simulink model "sl2ge_hyperloop"  (R2014a)
settings: Solver=FixedStepDiscrete  StartTime=startTime  StopTime=stopTime  FixedStep=0.025  MaxStep=0.1  RelTol=1e-3
values from neighbouring files (symbols this model uses):
  dactOffset = 0    [main_sl2ge.m]
  latOffset = offsetNSinMeters/110958.98    (= 0.0001802467903)    [main_sl2ge.m]
  pillarSpacing = 30    [main_sl2ge.m]
  startTime = 0    [main_sl2ge.m]    (also in sl2ge_multiple.m = evalin('base','startTime'))
  stopTime = logsout.getElement('dact').Values.Time(end)    [main_sl2ge.m]
undefined symbols (not defined in the file or in its folder): camHt_1LVal, camHt_1UVal, Chassis, getLOatTime, logsout, numPillars, sigbuilder_block, z_accel, z_dist, z_elevTube, z_height
undefined symbols (not defined in the file): camHt_1LTh, camHt_1UTh, camHt_2LTh, camHt_2UTh
libraries: simulink x10, realtime_pacer_lib x1, vrlib x1
settings Model: Creator=Administrator  LastModifiedBy=mbrauer
settings DataIOCC: SignalLoggingSaveFormat=ModelDataLogs  SignalLogging=off
settings OptimizationCC: ExpressionDepthLimit=2147483647
settings DebuggingCC: UnderspecifiedInitializationDetection=Classic  InheritedTsInSrcMsg=none  FcnCallInpInsideContextMsg=EnableAllAsWarning  StateNameClashWarn=warning
settings RTWCC: ProcessScript=grt_make_rtw_hook

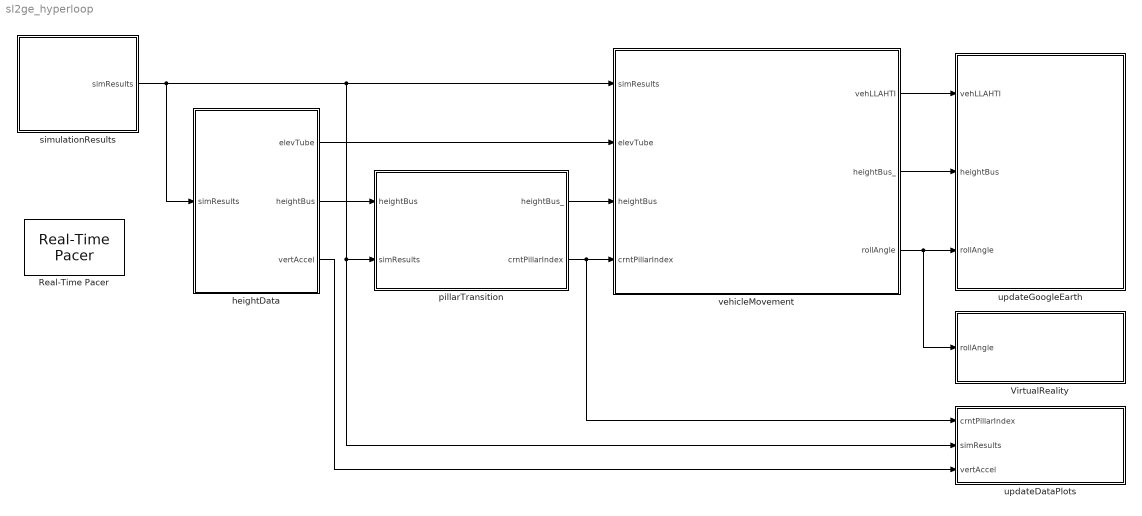
== system sl2ge_hyperloop ==
  Real-Time Pacer : realtime_pacer_lib/Real-Time Pacer  simTimePerRealTime=0.125
  VirtualReality : Subsystem
  heightData : Subsystem
  pillarTransition : Subsystem
  simulationResults : Subsystem
  updateDataPlots : Subsystem
  updateGoogleEarth : Subsystem
  vehicleMovement : Subsystem
  wires:
  heightData/1(elevTube) -> vehicleMovement/2(elevTube)
  pillarTransition/2(crntPillarIndex) -> vehicleMovement/4(crntPillarIndex), updateDataPlots/1(crntPillarIndex)
  vehicleMovement/3(rollAngle) -> updateGoogleEarth/3(rollAngle), VirtualReality/1(rollAngle)
  heightData/3(vertAccel) -> updateDataPlots/3(vertAccel)
  heightData/2(heightBus) -> pillarTransition/1(heightBus)
  pillarTransition/1(heightBus_) -> vehicleMovement/3(heightBus)
  vehicleMovement/2(heightBus_) -> updateGoogleEarth/2(heightBus)
  vehicleMovement/1(vehLLAHTI) -> updateGoogleEarth/1(vehLLAHTI)
  simulationResults/1(simResults) -> vehicleMovement/1(simResults), updateDataPlots/2(simResults), pillarTransition/2(simResults), heightData/1(simResults)

== system sl2ge_hyperloop/VirtualReality ==
  rollAngle : Inport
  CenterOfRotation : Constant  Value=[-1.54/2 sqrt(Chassis.TubeRadius^2-(1.54/2)^2) 0]'  SampleTime=-1
  Constant : Constant  Value=[0 0 1]'  SampleTime=-1
  Gain6 : Gain  Gain=-1
  VR Sink : vrlib/VR Sink  InstantiateOnLoad=on  SampleTime=-1  ViewEnable=on  RemoteChange=off  RemoteView=off  FieldsWritten=HyperPod.center.3.1.1.double#HyperPod.rotation.4.1.1.double  WorldFileName=hyperLoopPod3DTubeIso.wrl  WorldDescription=Simulink 3D Animation : Front View of Pod  AutoView=off  VideoDimensions=[]  AllowVariableSize=off
  Vector Concatenate1 : Concatenate
  wires:
  Gain6/1 -> Vector Concatenate1/2
  Constant/1 -> Vector Concatenate1/1
  CenterOfRotation/1 -> VR Sink/1
  Vector Concatenate1/1 -> VR Sink/2
  rollAngle/1 -> Gain6/1

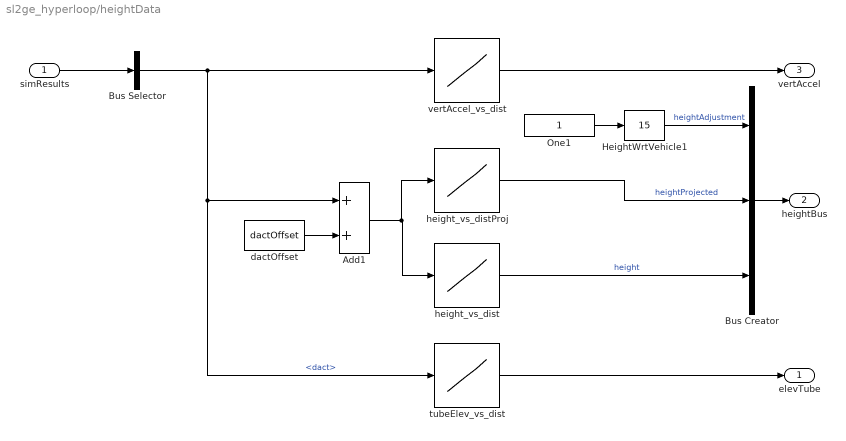
== system sl2ge_hyperloop/heightData ==
  simResults : Inport
  Add1 : Sum
  Bus Creator : BusCreator  Inputs=3
  Bus Selector : BusSelector  OutputSignals=dact
  HeightWrtVehicle1 : simulink/Math Operations/Slider Gain  low=-10  gain=15  high=30
  One1 : Constant  VectorParams1D=off
  dactOffset : Constant  Value=dactOffset
  height_vs_dist : Lookup_n-D  NumberOfTableDimensions=1  BreakpointsForDimension1=z_dist  BeginIndexSearchUsingPreviousIndexResult=on  Table=z_height  ExtrapMethod=Clip  InternalRulePriority=Speed  RndMeth=Simplest  InputSameDT=on
  height_vs_distProj : Lookup_n-D  NumberOfTableDimensions=1  BreakpointsForDimension1=z_dist-200  BeginIndexSearchUsingPreviousIndexResult=on  Table=z_height  ExtrapMethod=Clip  UseLastTableValue=on  InternalRulePriority=Speed  RndMeth=Simplest  InputSameDT=on
  tubeElev_vs_dist : Lookup_n-D  NumberOfTableDimensions=1  BreakpointsForDimension1=z_dist  BeginIndexSearchUsingPreviousIndexResult=on  Table=z_elevTube  InternalRulePriority=Speed  RndMeth=Simplest  InputSameDT=on
  vertAccel_vs_dist : Lookup_n-D  NumberOfTableDimensions=1  BreakpointsForDimension1=z_dist  BeginIndexSearchUsingPreviousIndexResult=on  Table=z_accel  ExtrapMethod=Clip  UseLastTableValue=on  InternalRulePriority=Speed  RndMeth=Simplest  InputSameDT=on
  elevTube : Outport
  heightBus : Outport  Port=2
  vertAccel : Outport  Port=3
  wires:
  height_vs_distProj/1 -> Bus Creator/2  "heightProjected"
  vertAccel_vs_dist/1 -> vertAccel/1
  height_vs_dist/1 -> Bus Creator/3  "height"
  tubeElev_vs_dist/1 -> elevTube/1
  Bus Selector/1 -> vertAccel_vs_dist/1, tubeElev_vs_dist/1, Add1/1  "<dact>"
  dactOffset/1 -> Add1/2
  Add1/1 -> height_vs_distProj/1, height_vs_dist/1
  One1/1 -> HeightWrtVehicle1/1
  HeightWrtVehicle1/1 -> Bus Creator/1  "heightAdjustment"
  Bus Creator/1 -> heightBus/1
  simResults/1 -> Bus Selector/1

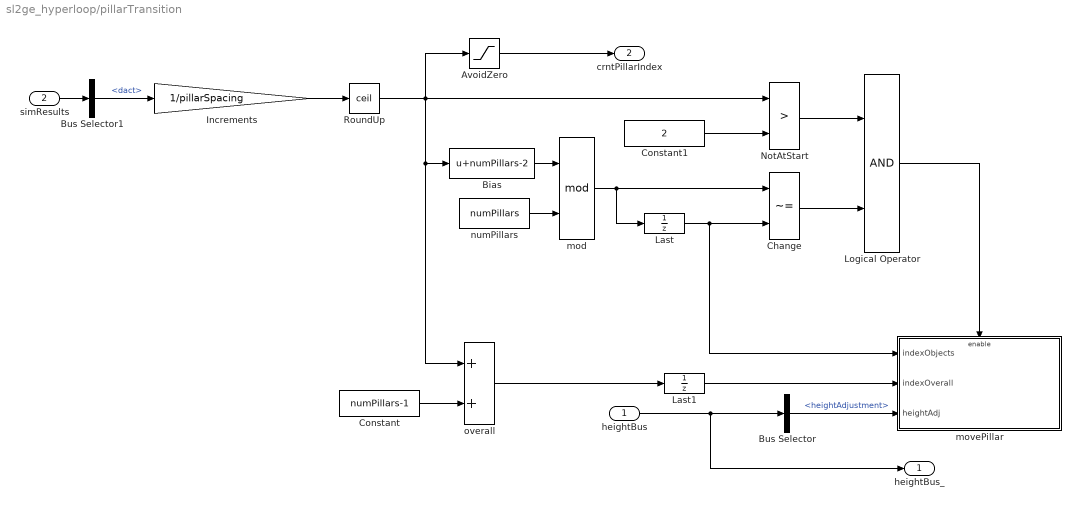
== system sl2ge_hyperloop/pillarTransition ==
  heightBus : Inport
  simResults : Inport  Port=2
  AvoidZero : Saturate  UpperLimit=inf  LowerLimit=1
  Bias : Bias  Bias=numPillars-2
  Bus Selector : BusSelector  OutputSignals=heightAdjustment
  Bus Selector1 : BusSelector  OutputSignals=dact
  Change : RelationalOperator  Operator=~=  OutDataTypeStr=boolean
  Constant : Constant  Value=numPillars-1
  Constant1 : Constant  Value=2
  Increments : Gain  Gain=1/pillarSpacing
  Last : UnitDelay  SampleTime=-1
  Last1 : UnitDelay  InitialCondition=1  SampleTime=-1
  Logical Operator : Logic  AllPortsSameDT=off  OutDataTypeStr=boolean
  NotAtStart : RelationalOperator  Operator=>  OutDataTypeStr=boolean
  RoundUp : Rounding  Operator=ceil
  mod : Math  Operator=mod  SaturateOnIntegerOverflow=on
  movePillar : Subsystem  TreatAsAtomicUnit=on
  numPillars : Constant  Value=numPillars
  overall : Sum
  heightBus_ : Outport
  crntPillarIndex : Outport  Port=2
  wires:
  Bus Selector1/1 -> Increments/1  "<dact>"
  Increments/1 -> RoundUp/1
  mod/1 -> Change/1, Last/1
  numPillars/1 -> mod/2
  Last/1 -> movePillar/1(indexObjects), Change/2
  overall/1 -> Last1/1
  Constant/1 -> overall/2
  Change/1 -> Logical Operator/2
  NotAtStart/1 -> Logical Operator/1
  Constant1/1 -> NotAtStart/2
  Logical Operator/1 -> movePillar/Enable
  Bias/1 -> mod/1
  RoundUp/1 -> AvoidZero/1, overall/1, Bias/1, NotAtStart/1
  Last1/1 -> movePillar/2(indexOverall)
  AvoidZero/1 -> crntPillarIndex/1
  heightBus/1 -> Bus Selector/1, heightBus_/1
  Bus Selector/1 -> movePillar/3(heightAdj)  "<heightAdjustment>"
  simResults/1 -> Bus Selector1/1

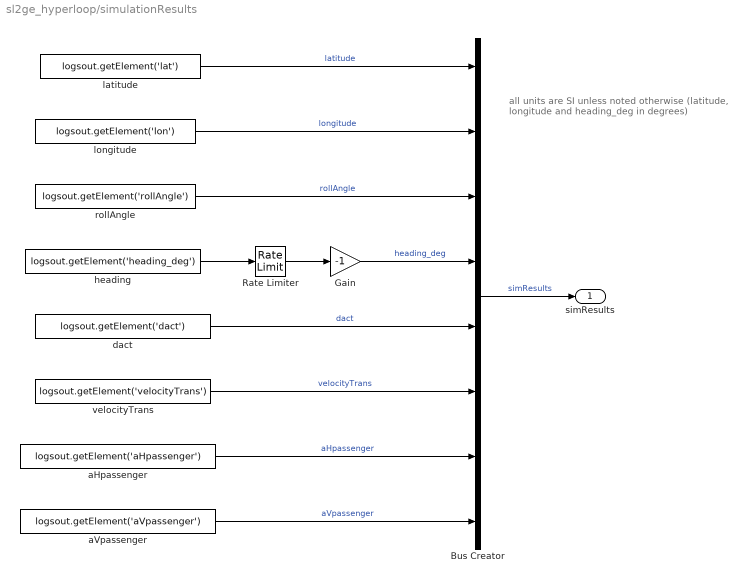
== system sl2ge_hyperloop/simulationResults ==
  note: all units are SI unless noted otherwise
      | (latitude, longitude and heading_deg in degrees)
  Bus Creator : BusCreator  Inputs=8
  Gain : Gain  Gain=-1
  Rate Limiter : RateLimiter  RisingSlewLimit=5  FallingSlewLimit=-5  SampleTimeMode=inherited  InitialCondition=getLOatTime(logsout, 'heading_deg', startTime)
  aHpassenger : FromWorkspace  VariableName=logsout.getElement('aHpassenger')
  aVpassenger : FromWorkspace  VariableName=logsout.getElement('aVpassenger')
  dact : FromWorkspace  VariableName=logsout.getElement('dact')
  heading : FromWorkspace  VariableName=logsout.getElement('heading_deg')
  latitude : FromWorkspace  VariableName=logsout.getElement('lat')
  longitude : FromWorkspace  VariableName=logsout.getElement('lon')
  rollAngle : FromWorkspace  VariableName=logsout.getElement('rollAngle')
  velocityTrans : FromWorkspace  VariableName=logsout.getElement('velocityTrans')
  simResults : Outport
  wires:
  Rate Limiter/1 -> Gain/1
  heading/1 -> Rate Limiter/1
  latitude/1 -> Bus Creator/1  "latitude"
  longitude/1 -> Bus Creator/2  "longitude"
  rollAngle/1 -> Bus Creator/3  "rollAngle"
  Gain/1 -> Bus Creator/4  "heading_deg"
  aHpassenger/1 -> Bus Creator/7  "aHpassenger"
  velocityTrans/1 -> Bus Creator/6  "velocityTrans"
  aVpassenger/1 -> Bus Creator/8  "aVpassenger"
  dact/1 -> Bus Creator/5  "dact"
  Bus Creator/1 -> simResults/1  "simResults"

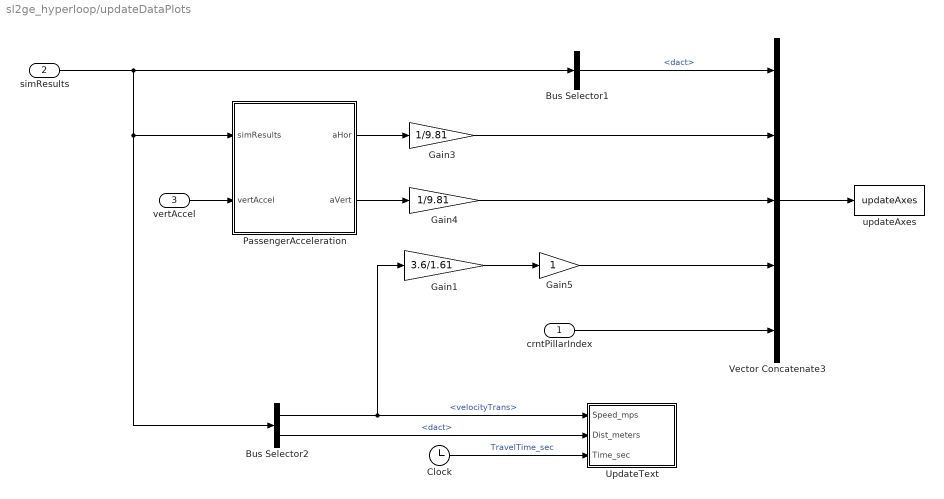
== system sl2ge_hyperloop/updateDataPlots ==
  crntPillarIndex : Inport
  simResults : Inport  Port=2
  vertAccel : Inport  Port=3
  Bus Selector1 : BusSelector  OutputSignals=dact
  Bus Selector2 : BusSelector  OutputSignals=velocityTrans,dact
  Clock : Clock
  Gain1 : Gain  Gain=3.6/1.61
  Gain3 : Gain  Gain=1/9.81
  Gain4 : Gain  Gain=1/9.81
  Gain5 : Gain
  PassengerAcceleration : Subsystem
  UpdateText : Subsystem
  Vector Concatenate3 : Concatenate  NumInputs=5  Mode=Multidimensional array  ConcatenateDimension=2
  updateAxes : MATLABFcn  MATLABFcn=updateAxes  OutputDimensions=0
  wires:
  Gain5/1 -> Vector Concatenate3/4
  Vector Concatenate3/1 -> updateAxes/1
  Gain3/1 -> Vector Concatenate3/2
  Gain4/1 -> Vector Concatenate3/3
  Gain1/1 -> Gain5/1
  Bus Selector2/1 -> Gain1/1, UpdateText/1(Speed_mps)  "<velocityTrans>"
  crntPillarIndex/1 -> Vector Concatenate3/5
  Bus Selector1/1 -> Vector Concatenate3/1  "<dact>"
  Clock/1 -> UpdateText/3(Time_sec)  "TravelTime_sec"
  PassengerAcceleration/1(aHor) -> Gain3/1
  PassengerAcceleration/2(aVert) -> Gain4/1
  vertAccel/1 -> PassengerAcceleration/2(vertAccel)
  simResults/1 -> PassengerAcceleration/1(simResults), Bus Selector2/1, Bus Selector1/1
  Bus Selector2/2 -> UpdateText/2(Dist_meters)  "<dact>"

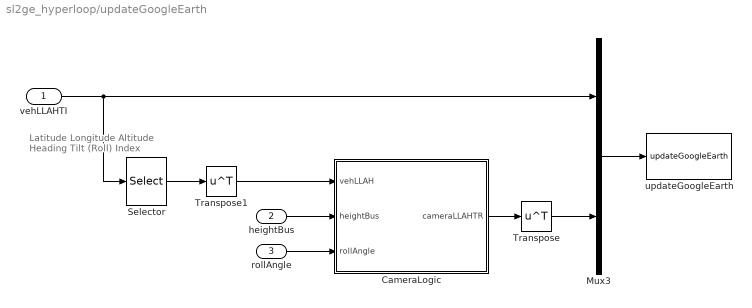
== system sl2ge_hyperloop/updateGoogleEarth ==
  note: Latitude
      | Longitude
      | Altitude
      | Heading
      | Tilt (Roll)
      | Index
  vehLLAHTI : Inport
  heightBus : Inport  Port=2
  rollAngle : Inport  Port=3
  CameraLogic : Subsystem
  Mux3 : Mux  Inputs=2
  Selector : Selector  InputPortWidth=6  Indices=[1 2 3 4]
  Transpose : Math  Operator=transpose  SaturateOnIntegerOverflow=on
  Transpose1 : Math  Operator=transpose  SaturateOnIntegerOverflow=on
  updateGoogleEarth : MATLABFcn  MATLABFcn=updateGoogleEarth  OutputDimensions=0
  wires:
  Selector/1 -> Transpose1/1
  Transpose/1 -> Mux3/2
  vehLLAHTI/1 -> Selector/1, Mux3/1
  Mux3/1 -> updateGoogleEarth/1
  Transpose1/1 -> CameraLogic/1(vehLLAH)
  heightBus/1 -> CameraLogic/2(heightBus)
  rollAngle/1 -> CameraLogic/3(rollAngle)
  CameraLogic/1(cameraLLAHTR) -> Transpose/1

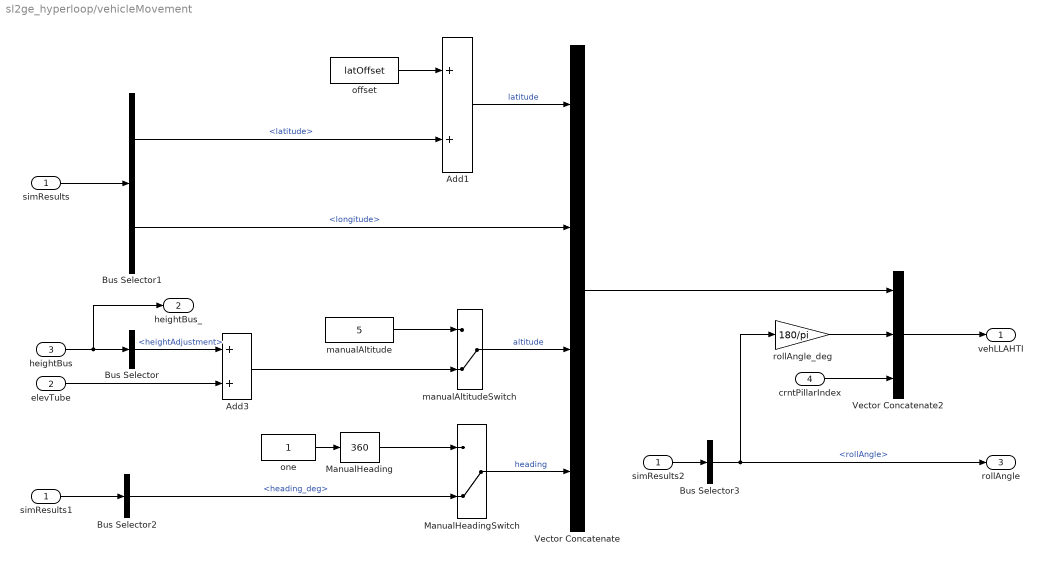
== system sl2ge_hyperloop/vehicleMovement ==
  simResults : Inport
  elevTube : Inport  Port=2
  heightBus : Inport  Port=3
  crntPillarIndex : Inport  Port=4
  Add1 : Sum
  Add3 : Sum
  Bus Selector : BusSelector  OutputSignals=heightAdjustment
  Bus Selector1 : BusSelector  OutputSignals=latitude,longitude
  Bus Selector2 : BusSelector  OutputSignals=heading_deg
  Bus Selector3 : BusSelector  OutputSignals=rollAngle
  ManualHeading : simulink/Math Operations/Slider Gain  low=-360  gain=360  high=360
  ManualHeadingSwitch : ManualSwitch  CurrentSetting=0
  Vector Concatenate : Concatenate  NumInputs=4  Mode=Multidimensional array  ConcatenateDimension=2
  Vector Concatenate2 : Concatenate  NumInputs=3  ConcatenateDimension=2
  manualAltitude : Constant  Value=5  VectorParams1D=off
  manualAltitudeSwitch : ManualSwitch  CurrentSetting=0
  offset : Constant  Value=latOffset  VectorParams1D=off
  one : Constant  VectorParams1D=off
  rollAngle_deg : Gain  Gain=180/pi
  simResults1 : InportShadow
  simResults2 : InportShadow
  vehLLAHTI : Outport
  heightBus_ : Outport  Port=2
  rollAngle : Outport  Port=3
  wires:
  Vector Concatenate2/1 -> vehLLAHTI/1
  rollAngle_deg/1 -> Vector Concatenate2/2
  Vector Concatenate/1 -> Vector Concatenate2/1
  Add3/1 -> manualAltitudeSwitch/2
  heightBus/1 -> Bus Selector/1, heightBus_/1
  manualAltitudeSwitch/1 -> Vector Concatenate/3  "altitude"
  manualAltitude/1 -> manualAltitudeSwitch/1
  Bus Selector2/1 -> ManualHeadingSwitch/2  "<heading_deg>"
  one/1 -> ManualHeading/1
  ManualHeadingSwitch/1 -> Vector Concatenate/4  "heading"
  Bus Selector1/2 -> Vector Concatenate/2  "<longitude>"
  crntPillarIndex/1 -> Vector Concatenate2/3
  Bus Selector1/1 -> Add1/2  "<latitude>"
  Add1/1 -> Vector Concatenate/1  "latitude"
  offset/1 -> Add1/1
  Bus Selector/1 -> Add3/1  "<heightAdjustment>"
  elevTube/1 -> Add3/2
  ManualHeading/1 -> ManualHeadingSwitch/1
  simResults/1 -> Bus Selector1/1
  simResults1/1 -> Bus Selector2/1
  simResults2/1 -> Bus Selector3/1
  Bus Selector3/1 -> rollAngle_deg/1, rollAngle/1  "<rollAngle>"

== system sl2ge_hyperloop/pillarTransition/movePillar ==
  indexObjects : Inport
  indexOverall : Inport  Port=2
  heightAdj : Inport  Port=3
  Enable : EnablePort  StatesWhenEnabling=reset
  Mux : Mux  Inputs=3
  updatePillar : MATLABFcn  MATLABFcn=updatePillars  OutputDimensions=0
  wires:
  indexObjects/1 -> Mux/1
  indexOverall/1 -> Mux/2
  Mux/1 -> updatePillar/1
  heightAdj/1 -> Mux/3

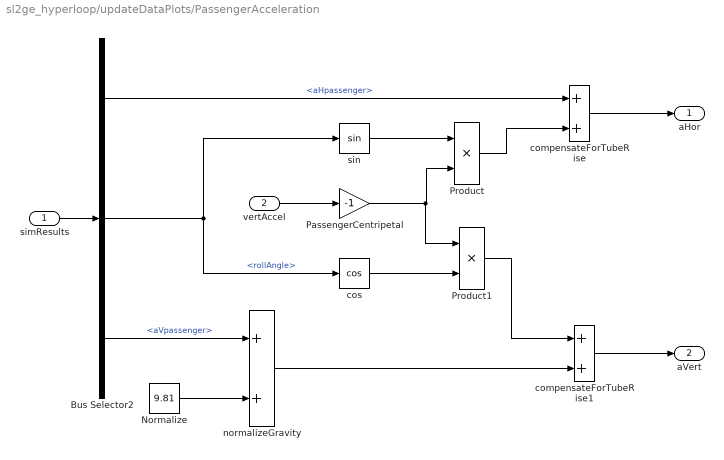
== system sl2ge_hyperloop/updateDataPlots/PassengerAcceleration ==
  simResults : Inport
  vertAccel : Inport  Port=2
  Bus Selector2 : BusSelector  OutputSignals=aHpassenger,rollAngle,aVpassenger
  Normalize : Constant  Value=9.81
  PassengerCentripetal : Gain  Gain=-1
  Product : Product
  Product1 : Product
  compensateForTubeRise : Sum
  compensateForTubeRise1 : Sum
  cos : Trigonometry  Operator=cos
  normalizeGravity : Sum
  sin : Trigonometry
  aHor : Outport
  aVert : Outport  Port=2
  wires:
  Bus Selector2/3 -> normalizeGravity/1  "<aVpassenger>"
  Normalize/1 -> normalizeGravity/2
  Bus Selector2/2 -> cos/1, sin/1  "<rollAngle>"
  sin/1 -> Product/1
  cos/1 -> Product1/2
  vertAccel/1 -> PassengerCentripetal/1
  compensateForTubeRise/1 -> aHor/1
  Bus Selector2/1 -> compensateForTubeRise/1  "<aHpassenger>"
  compensateForTubeRise1/1 -> aVert/1
  normalizeGravity/1 -> compensateForTubeRise1/2
  Product1/1 -> compensateForTubeRise1/1
  Product/1 -> compensateForTubeRise/2
  PassengerCentripetal/1 -> Product1/1, Product/2
  simResults/1 -> Bus Selector2/1

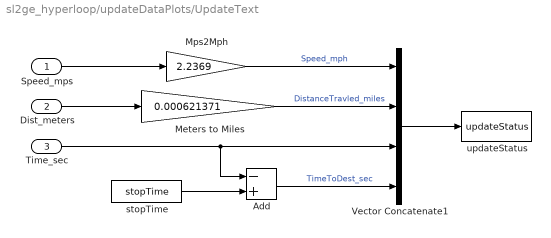
== system sl2ge_hyperloop/updateDataPlots/UpdateText ==
  Speed_mps : Inport
  Dist_meters : Inport  Port=2
  Time_sec : Inport  Port=3
  Add : Sum  Inputs=-+
  Meters to Miles : Gain  Gain=0.000621371
  Mps2Mph : Gain  Gain=2.2369
  Vector Concatenate1 : Concatenate  NumInputs=4  Mode=Multidimensional array  ConcatenateDimension=2
  stopTime : Constant  Value=stopTime
  updateStatus : MATLABFcn  MATLABFcn=updateStatus  OutputDimensions=0
  wires:
  Dist_meters/1 -> Meters to Miles/1
  Vector Concatenate1/1 -> updateStatus/1
  Mps2Mph/1 -> Vector Concatenate1/1  "Speed_mph"
  Meters to Miles/1 -> Vector Concatenate1/2  "DistanceTravled_miles"
  Time_sec/1 -> Vector Concatenate1/3, Add/1
  stopTime/1 -> Add/2
  Add/1 -> Vector Concatenate1/4  "TimeToDest_sec"
  Speed_mps/1 -> Mps2Mph/1

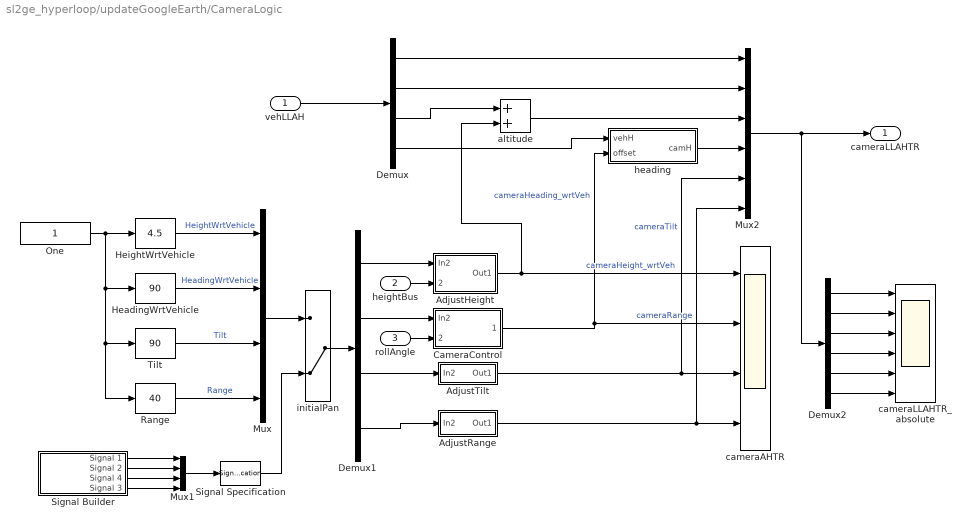
== system sl2ge_hyperloop/updateGoogleEarth/CameraLogic ==
  vehLLAH : Inport
  heightBus : Inport  Port=2
  rollAngle : Inport  Port=3
  AdjustHeight : Subsystem
  AdjustRange : Subsystem
  AdjustTilt : Subsystem
  CameraControl : Subsystem
  Demux : Demux
  Demux1 : Demux
  Demux2 : Demux  Outputs=6
  HeadingWrtVehicle : simulink/Math Operations/Slider Gain  low=65  gain=90  high=115
  HeightWrtVehicle : simulink/Math Operations/Slider Gain  low=0  gain=4.5  high=30
  Mux : Mux
  Mux1 : Mux
  Mux2 : Mux  Inputs=6
  One : Constant  VectorParams1D=off
  Range : simulink/Math Operations/Slider Gain  low=20  gain=40  high=60
  Signal Builder : Subsystem  Tag=STV Subsys  LoadFcn=sigbuilder_block('load');  StartFcn=sigbuilder_block('start');  StopFcn=sigbuilder_block('stop');  ClipboardFcn=sigbuilder_block('clipboard');  mask(Sigbuilder block){}
      mask help: Simulink:masks:SigbuilderBlock_MD
      mask init:
      | if ~strcmp(get_param(bdroot(gcbh),'SimulationStatus'),'stopped') tuvar = sigbuilder_block('maskInit'); end
      settings: CopyFcn=sigbuilder_block('copy');  DeleteFcn=sigbuilder_block('delete');  ModelCloseFcn=sigbuilder_block('modelClose');  PreSaveFcn=sigbuilder_block('preSave');  PauseFcn=sigbuilder_block('pause');  ContinueFcn=sigbuilder_block('continue');  NameChangeFcn=sigbuilder_block('namechange');  OpenFcn=sigbuilder_block('open',[679.5 100.5 550.5 399.75 ]);  CloseFcn=sigbuilder_block('close');
      mask Display: plot(0, 0, 100, 100,[2, 2, 32, 32, 2], [68, 8, 8, 68, 68],[32, 2], [38, 38], [32, 19, 2],[53, 60, 44], [32, 17, 17, 2],[16, 16, 31, 31]);txt = getActiveGroup(gcbh);text(2, 100, txt,'verticalAlignment', 'top');
  Signal Specification : SignalSpecification  SampleTime=0.025
  Tilt : simulink/Math Operations/Slider Gain  low=0  gain=90  high=180
  altitude : Sum
  cameraAHTR : Scope  NumInputPorts=4
      settings: YMin=1.8~35~90~15  YMax=3~70~90~15
  cameraLLAHTR_absolute : Scope  NumInputPorts=6
      settings: YMin=-5~-5~-5~-5~-5~-5  YMax=5~5~5~5~5~5  SaveName=ScopeData2
  heading : Subsystem
  initialPan : ManualSwitch  CurrentSetting=0
  cameraLLAHTR : Outport
  wires:
  Mux2/1 -> cameraLLAHTR/1, Demux2/1
  vehLLAH/1 -> Demux/1
  Demux/1 -> Mux2/1
  Range/1 -> Mux/4  "Range"
  Demux1/2 -> CameraControl/1(In2)
  HeightWrtVehicle/1 -> Mux/1  "HeightWrtVehicle"
  AdjustRange/1(Out1) -> Mux2/6, cameraAHTR/4  "cameraRange"
  Mux/1 -> initialPan/1
  HeadingWrtVehicle/1 -> Mux/2  "HeadingWrtVehicle"
  Demux/3 -> altitude/1
  One/1 -> HeightWrtVehicle/1, Range/1, Tilt/1, HeadingWrtVehicle/1
  Demux/2 -> Mux2/2
  AdjustHeight/1(Out1) -> cameraAHTR/1, altitude/2  "cameraHeight_wrtVeh"
  Tilt/1 -> Mux/3  "Tilt"
  Demux1/3 -> AdjustTilt/1(In2)
  initialPan/1 -> Demux1/1
  Demux1/1 -> AdjustHeight/1(In2)
  Demux1/4 -> AdjustRange/1(In2)
  Demux2/6 -> cameraLLAHTR_absolute/6
  Signal Builder/3(Signal 4) -> Mux1/3
  Signal Builder/1(Signal 1) -> Mux1/1
  Mux1/1 -> Signal Specification/1
  Signal Specification/1 -> initialPan/2
  Demux2/5 -> cameraLLAHTR_absolute/5
  Demux2/1 -> cameraLLAHTR_absolute/1
  Signal Builder/4(Signal 3) -> Mux1/4
  CameraControl/1(heading) -> cameraAHTR/2, heading/2(offset)  "cameraHeading_wrtVeh"
  altitude/1 -> Mux2/3
  Signal Builder/2(Signal 2) -> Mux1/2
  Demux2/2 -> cameraLLAHTR_absolute/2
  Demux2/4 -> cameraLLAHTR_absolute/4
  Demux2/3 -> cameraLLAHTR_absolute/3
  rollAngle/1 -> CameraControl/2(rollAngle)
  AdjustTilt/1(Out1) -> Mux2/5, cameraAHTR/3  "cameraTilt"
  heightBus/1 -> AdjustHeight/2(heightBus)
  Demux/4 -> heading/1(vehH)
  heading/1(camH) -> Mux2/4

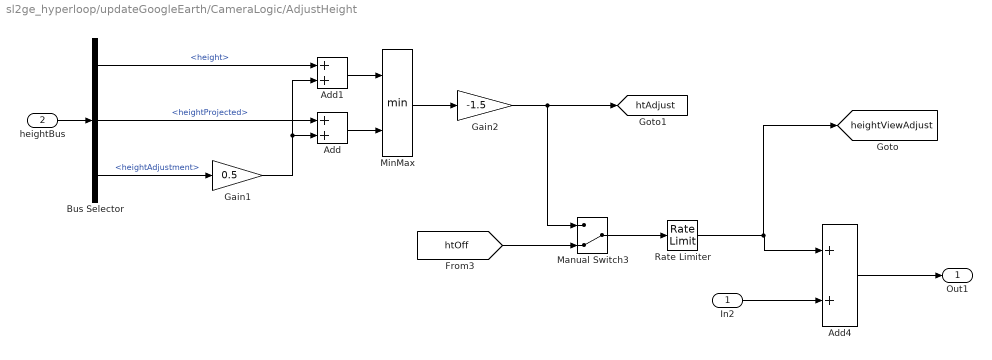
== system sl2ge_hyperloop/updateGoogleEarth/CameraLogic/AdjustHeight ==
  In2 : Inport
  heightBus : Inport  Port=2
  Add : Sum
  Add1 : Sum
  Add4 : Sum
  Bus Selector : BusSelector  OutputSignals=height,heightProjected,heightAdjustment
  Gain1 : Gain  Gain=0.5
  Gain2 : Gain  Gain=-1.5
  Manual Switch3 : ManualSwitch  CurrentSetting=0
  MinMax : MinMax  Inputs=2
  Rate Limiter : RateLimiter  RisingSlewLimit=5  FallingSlewLimit=-5  SampleTimeMode=inherited
  Out1 : Outport
  tag scope: heightViewAdjust=global, htAdjust=global
  wires:
  Add4/1 -> Out1/1
  [htOff] -> Manual Switch3/2
  MinMax/1 -> Gain2/1
  Manual Switch3/1 -> Rate Limiter/1
  In2/1 -> Add4/2
  Add/1 -> MinMax/2
  Rate Limiter/1 -> [heightViewAdjust], Add4/1
  Bus Selector/2 -> Add/1  "<heightProjected>"
  Gain1/1 -> Add1/2, Add/2
  Add1/1 -> MinMax/1
  Gain2/1 -> Manual Switch3/1, [htAdjust]
  heightBus/1 -> Bus Selector/1
  Bus Selector/1 -> Add1/1  "<height>"
  Bus Selector/3 -> Gain1/1  "<heightAdjustment>"

== system sl2ge_hyperloop/updateGoogleEarth/CameraLogic/AdjustRange ==
  In2 : Inport
  1-D Lookup Table : Lookup_n-D  NumberOfTableDimensions=1  BreakpointsForDimension1=[0 45 90]  Table=[120 80 0]  ExtrapMethod=Clip  UseLastTableValue=on  InternalRulePriority=Speed  RndMeth=Simplest  InputSameDT=on
  Add4 : Sum
  Gain : Gain
  Ground1 : Ground
  Manual Switch3 : ManualSwitch
  Out1 : Outport
  wires:
  Gain/1 -> Manual Switch3/1
  Add4/1 -> Out1/1
  Ground1/1 -> Manual Switch3/2
  [Tilt] -> 1-D Lookup Table/1
  Manual Switch3/1 -> Add4/1
  In2/1 -> Add4/2
  1-D Lookup Table/1 -> Gain/1

== system sl2ge_hyperloop/updateGoogleEarth/CameraLogic/AdjustTilt ==
  In2 : Inport
  1-D Lookup Table : Lookup_n-D  NumberOfTableDimensions=1  BreakpointsForDimension1=[0 2 30 60]  Table="[0  -5 -50 -80]"  InternalRulePriority=Speed  RndMeth=Simplest  InputSameDT=on
  Add4 : Sum
  Gain : Gain
  Ground1 : Ground
  Manual Switch3 : ManualSwitch
  Out1 : Outport
  tag scope: Tilt=global
  wires:
  1-D Lookup Table/1 -> Gain/1
  In2/1 -> Add4/2
  Manual Switch3/1 -> Add4/1
  [heightViewAdjust] -> 1-D Lookup Table/1
  Ground1/1 -> Manual Switch3/2
  Add4/1 -> [Tilt], Out1/1
  Gain/1 -> Manual Switch3/1

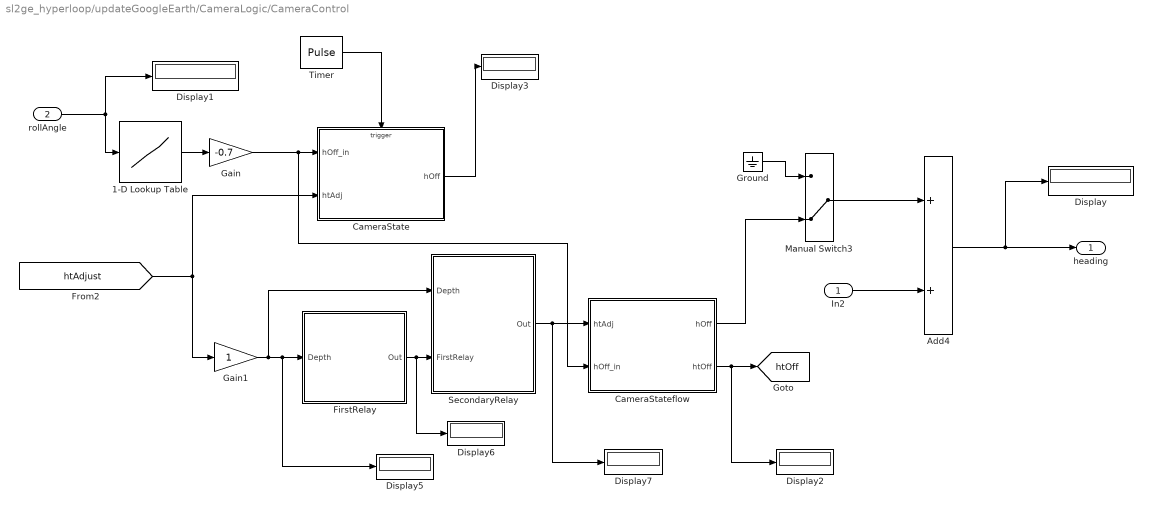
== system sl2ge_hyperloop/updateGoogleEarth/CameraLogic/CameraControl ==
  In2 : Inport
  rollAngle : Inport  Port=2
  1-D Lookup Table : Lookup_n-D  NumberOfTableDimensions=1  BreakpointsForDimension1=[-0.5 0 0.5]  Table=[-30 0 30]  InternalRulePriority=Speed  RndMeth=Simplest  InputSameDT=on
  Add4 : Sum
  CameraState : Stateflow chart  TreatAsAtomicUnit=on
  CameraStateflow : Stateflow chart  TreatAsAtomicUnit=on
  Display{,1..3,5..7} (7 alike) : Display
  FirstRelay : Subsystem  mask{UL=camHt_1UTh, LL=camHt_1LTh, UValue=camHt_1UVal, LValue=camHt_1LVal}
      mask prompts: UL "Upper Threshold"; LL "Lower Threshold"; UValue "Upper Value"; LValue "Lower Value"
  Gain : Gain  Gain=-0.7
  Gain1 : Gain
  Ground : Ground
  Manual Switch3 : ManualSwitch  CurrentSetting=0
  SecondaryRelay : Subsystem  mask{UL=camHt_2UTh, LL=camHt_2LTh}
      mask prompts: UL "Upper Threshold"; LL "Lower Threshold"
  Timer : DiscretePulseGenerator  PulseType=Time based  Period=1  PulseWidth=50
  heading : Outport
  tag scope: htOff=global
  wires:
  Add4/1 -> Display/1, heading/1
  CameraStateflow/1(hOff) -> Manual Switch3/2
  rollAngle/1 -> 1-D Lookup Table/1, Display1/1
  In2/1 -> Add4/2
  1-D Lookup Table/1 -> Gain/1
  Timer/1 -> CameraState/Trigger
  CameraState/1(hOff) -> Display3/1
  Gain/1 -> CameraStateflow/2(hOff_in), CameraState/1(hOff_in)
  [htAdjust] -> Gain1/1, CameraState/2(htAdj)
  FirstRelay/1(Out) -> Display6/1, SecondaryRelay/2(FirstRelay)
  Gain1/1 -> Display5/1, FirstRelay/1(Depth), SecondaryRelay/1(Depth)
  SecondaryRelay/1(Out) -> Display7/1, CameraStateflow/1(htAdj)
  Manual Switch3/1 -> Add4/1
  CameraStateflow/2(htOff) -> Display2/1, [htOff]
  Ground/1 -> Manual Switch3/1

== system sl2ge_hyperloop/updateGoogleEarth/CameraLogic/Signal Builder ==
  Demux : Demux  Tag=STV Demux
  FromWs : FromWorkspace  Tag=STV FromWs  VariableName=tuvar  SampleTime=0
      SigBuilderData=|
      | common.afterFinalStr = 'Extrapolate'
      | common.sampleTime = 0
      | dataSet.timeRange = [0 15]
      | dataSet.name = 'Group 1'
      | sbobj.Groups.Name = 'Group 1'
      | sbobj.Groups.Signals(1).Name = 'Signal 1'
      | sbobj.Groups.Signals(1).XData = [0 5.02 10 15]
      | sbobj.Groups.Signals(1).YData = [1.8 1.8 4.78 4.78]
      | sbobj.Groups.Signals(2).Name = 'Signal 2'
      | sbobj.Groups.Signals(2).XData = [0 1 5 10 15]
      | sbobj.Groups.Signals(2).YData = [84 84 60 90 90]
      | sbobj.Groups.Signals(3).Name = 'Signal 4'
      | sbobj.Groups.Signals(3).XData = [0 15]
      | sbobj.Groups.Signals(3).YData = [90 90]
      | sbobj.Groups.Signals(4).Name = 'Signal 3'
      | sbobj.Groups.Signals(4).XData = [0 5 10 15]
      | sbobj.Groups.Signals(4).YData = [15 15 40 40]
      | sbobj.Groups.TimeRange = [0 15]
  Signal 1 : Outport  Tag=STV Outport
  Signal 2 : Outport  Tag=STV Outport  Port=2
  Signal 4 : Outport  Tag=STV Outport  Port=3
  Signal 3 : Outport  Tag=STV Outport  Port=4
  wires:
  FromWs/1 -> Demux/1
  Demux/1 -> Signal 1/1
  Demux/2 -> Signal 2/1
  Demux/3 -> Signal 4/1
  Demux/4 -> Signal 3/1

== system sl2ge_hyperloop/updateGoogleEarth/CameraLogic/heading ==
  vehH : Inport
  offset : Inport  Port=2
  Ground : Ground
  Manual Switch : ManualSwitch
  Rate Limiter1 : RateLimiter  RisingSlewLimit=7.5  FallingSlewLimit=-7.5  SampleTimeMode=inherited  InitialCondition=getLOatTime(logsout, 'heading_deg', startTime)
  height : Sum
  camH : Outport
  wires:
  Ground/1 -> Manual Switch/2
  vehH/1 -> Manual Switch/1
  height/1 -> Rate Limiter1/1
  Manual Switch/1 -> height/1
  Rate Limiter1/1 -> camH/1
  offset/1 -> height/2

== system sl2ge_hyperloop/updateGoogleEarth/CameraLogic/CameraControl/FirstRelay ==
  Depth : Inport
  Constant : Constant  Value=UValue
  Constant1 : Constant  Value=LValue
  GreaterThan : simulink/Logic and Bit Operations/Compare To Constant  relop=>  const=UL  OutDataTypeStr=boolean
  LessThan : simulink/Logic and Bit Operations/Compare To Constant  relop=<  const=LL  OutDataTypeStr=boolean
  Relay : UnitDelay  SampleTime=-1
  Switch : Switch  Criteria=u2 > Threshold
  Switch1 : Switch  Criteria=u2 > Threshold
  Out : Outport
  wires:
  Switch1/1 -> Relay/1, Out/1
  Relay/1 -> Switch/3
  LessThan/1 -> Switch1/2
  Depth/1 -> LessThan/1, GreaterThan/1
  GreaterThan/1 -> Switch/2
  Switch/1 -> Switch1/3
  Constant/1 -> Switch/1
  Constant1/1 -> Switch1/1

== system sl2ge_hyperloop/updateGoogleEarth/CameraLogic/CameraControl/SecondaryRelay ==
  Depth : Inport
  FirstRelay : Inport  Port=2
  GreaterThan : simulink/Logic and Bit Operations/Compare To Constant  relop=>  const=UL  OutDataTypeStr=boolean
  LessThan : simulink/Logic and Bit Operations/Compare To Constant  relop=>=  const=LL  OutDataTypeStr=boolean
  Relay : UnitDelay  SampleTime=-1
  Switch : Switch  Criteria=u2 > Threshold
  Switch1 : Switch  Criteria=u2 > Threshold
  Out : Outport
  wires:
  GreaterThan/1 -> Switch/2
  Depth/1 -> Switch/1, LessThan/1, GreaterThan/1
  LessThan/1 -> Switch1/2
  FirstRelay/1 -> Switch1/3
  Relay/1 -> Switch/3
  Switch1/1 -> Out/1, Relay/1
  Switch/1 -> Switch1/1

== stateflow chart sl2ge_hyperloop/updateGoogleEarth/CameraLogic/CameraControl/CameraStateflow ==
  state Overhead
    state Overhead
      du: htOff=max(20,htAdj);
      hOff=hOff_in;
    state Delay
    (default) -> Overhead.Overhead
    Delay -> Overhead.Overhead [order 2] : [htAdj > camHt_1UVal]
    Overhead.Overhead -> Delay : [htAdj < camHt_1UVal]
  state Flat
    state PanRight
      en:hOff = -25;
      coinRight = false;
    state PanLeft
      en:hOff = 25;
      coinRight = true;
    state RearView
      entry: hOff = 0;
      htOff = camHt_1LVal;
    (default) -> RearView
    Flat.PanLeft -> RearView : after(6,sec)
    Flat.PanRight -> RearView : after(8,sec)
    RearView -> (junction 6) : after(2,sec)
    (junction 6) -> Flat.PanRight [order 1] : [coinRight]
    (junction 6) -> Flat.PanLeft [order 2]
  state Shallow
    state PanRight
      en:hOff = -25;
      coinRight = false;
    state PanLeft
      en:hOff = 25;
      coinRight = true;
    (default) -> (junction 73) : { htOff=camHt_1UVal;}
    (junction 73) -> Shallow.PanLeft [order 2]
    (junction 73) -> Shallow.PanRight [order 1] : [hOff<=0]
    Shallow.PanLeft -> Shallow.PanRight : after(10,sec)
    Shallow.PanRight -> Shallow.PanLeft : after(10,sec)
  (default) -> Flat : {coinRight=true;}
  Shallow -> Flat [order 1] : [htAdj <= camHt_1LVal]
  Flat -> Shallow : [htAdj > camHt_1LVal]
  Shallow -> Overhead [order 2] : [htAdj > camHt_1UVal]
  Delay -> Shallow [order 1] : after(1.5,sec)
  data: hOff output; coinRight local boolean =true; htAdj input; htOff output; camHt_1LVal parameter; camHt_1UVal parameter; hOff_in input

== stateflow chart sl2ge_hyperloop/updateGoogleEarth/CameraLogic/CameraControl/CameraState ==
  state PanLeft
    state Proportional
      en:hOff = 20;
    state ScanToFront
      du:
      hOff = 70;
    (default) -> PanLeft.Proportional
    PanLeft.Proportional -> PanLeft.ScanToFront : after(10,secs)
    PanLeft.ScanToFront -> PanLeft.Proportional : after(10,secs)
  state PanRight
    state Proportional
      en:hOff = -20;
    state ScanToFront
      du:
      hOff = -70;
    (default) -> PanRight.Proportional
    PanRight.Proportional -> PanRight.ScanToFront : after(10,secs)
    PanRight.ScanToFront -> PanRight.Proportional : after(10,secs)
  state Hover
    state HoverLeft
      en:hOff = 20;
      coinRight = true;
    state HoverRight
      en:hOff = -20;
      coinRight = false;
    state HoverOver
      entry: hOff = 0;
    (junction 6) -> HoverLeft [order 2]
    (junction 6) -> HoverRight [order 1] : [coinRight]
    HoverOver -> (junction 6) : after(2,secs)
    HoverLeft -> HoverOver : after(10,secs)
    HoverRight -> HoverOver : after(10,secs)
    (default) -> HoverOver
  state Overhead
    du: hOff=hOff_in;
  (default) -> Hover : {coinRight=true;}
  Hover -> PanRight [order 2] : [hOff_in<-10]
  Hover -> PanLeft [order 1] : [hOff_in>10]
  PanLeft -> HoverLeft [order 1] : [hOff_in<5]
  PanRight -> HoverRight [order 1] : [hOff_in>-5]
  PanLeft -> Overhead [order 2] : [htAdj > 3]
  Overhead -> Hover : [htAdj<1]
  Hover -> Overhead [order 3] : [htAdj > 3]
  PanRight -> Overhead [order 2] : [htAdj > 3]
  data: hOff output; hOff_in input; coinRight local boolean =true; htAdj input
  events: secs input RISING_EDGE_EVENT
